simulink model "Observer"  (Simulink 8.6)
settings: Solver=ode45  StartTime=0.0  StopTime=10.0  RelTol=1e-3
values from neighbouring files (symbols this model uses):
  c1 = 5    [Parameters.m]
  c2 = 5    [Parameters.m]
  c3 = 5    [Parameters.m]
  l1 = Prm(3)    [Coriolis.m]    (also in Inertia.m; P1.m; P2.m; Parameters.m = 0.4)
  l2 = Prm(4)    [Coriolis.m]    (also in Inertia.m; P1.m; P2.m; Parameters.m = 0.3)
  m1 = Prm(1)    [Coriolis.m]    (also in Inertia.m; P1.m; Parameters.m = 1.5; Psi.m)
  m2 = Prm(2)    [Coriolis.m]    (also in Inertia.m; P1.m; P2.m; Parameters.m = 1)
  q_0 = [0;0]    [Parameters.m]
  q_dot0 = [0;0]    [Parameters.m]
  q_hat0 = [0;0]    [Parameters.m]
  r_0 = 0    [Parameters.m]
  x_hat0 = [0;0]    [Parameters.m]
  xi_0 = [0;0]    [Parameters.m]
settings Model: Creator=TOSHIBA  LastModifiedBy=TOSHIBA
settings DataIOCC: SaveFormat=StructureWithTime  SignalLoggingSaveFormat=Dataset
settings OptimizationCC: ExpressionDepthLimit=128
settings DebuggingCC: UnderspecifiedInitializationDetection=Simplified  MergeDetectMultiDrivingBlocksExec=error  SolverPrmCheckMsg=none  FcnCallInpInsideContextMsg=EnableAllAsError  StateNameClashWarn=none
settings HardwareCC: ProdBitPerPointer=64  ProdLargestAtomicFloat=Float  ProdIntDivRoundTo=Zero  ProdEndianess=LittleEndian  ProdHWDeviceType=Specified
settings GRTTargetCC: GeneratePreprocessorConditionals=Use local settings  CombineOutputUpdateFcns=on  GRTInterface=off
settings ConfigComp: CovModelRefEnable=off

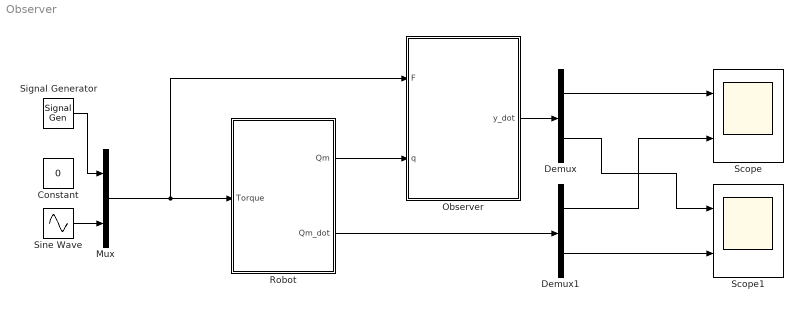
== system Observer ==
  Constant : Constant  Value=0
  Demux : Demux  Outputs=2
  Demux1 : Demux  Outputs=2
  Mux : Mux  Inputs=2
  Observer : Subsystem
  Robot : Subsystem
  Scope : Scope  NumInputPorts=2
  Scope1 : Scope  NumInputPorts=2
  Signal Generator : SignalGenerator  WaveForm=sawtooth  Amplitude=0.01  Frequency=pi  Units=rad/sec
  Sine Wave : Sin  Amplitude=0.001  Frequency=pi/1  SampleTime=0
  wires:
  Sine Wave/1 -> Mux/2
  Mux/1 -> Observer/1(F), Robot/1(Torque)
  Observer/1(y_dot) -> Demux/1
  Robot/2(Qm_dot) -> Demux1/1
  Demux/1 -> Scope/1
  Demux1/1 -> Scope/2
  Demux/2 -> Scope1/1
  Demux1/2 -> Scope1/2
  Robot/1(Qm) -> Observer/2(q)
  Signal Generator/1 -> Mux/1

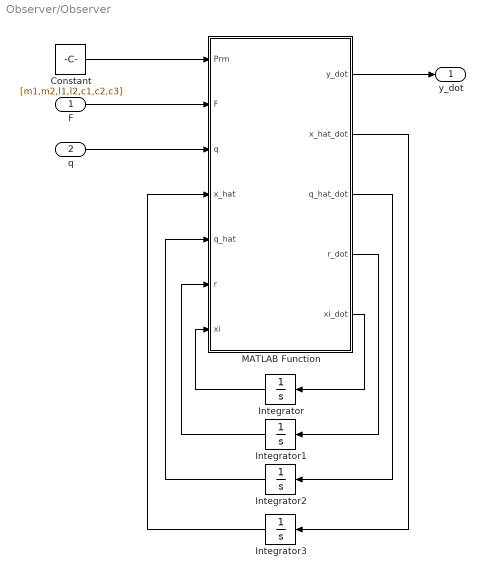
== system Observer/Observer ==
  F : Inport
  q : Inport  Port=2
  Constant : Constant  Value=[m1,m2,l1,l2,c1,c2,c3]
  Integrator : Integrator  InitialCondition=xi_0
  Integrator1 : Integrator  InitialCondition=r_0
  Integrator2 : Integrator  InitialCondition=q_hat0
  Integrator3 : Integrator  InitialCondition=x_hat0
  MATLAB Function : MATLAB Function  TreatAsAtomicUnit=on
  y_dot : Outport
  wires:
  F/1 -> MATLAB Function/2(F)
  q/1 -> MATLAB Function/3(q)
  Constant/1 -> MATLAB Function/1(Prm)
  MATLAB Function/5(xi_dot) -> Integrator/1
  Integrator/1 -> MATLAB Function/7(xi)
  Integrator1/1 -> MATLAB Function/6(r)
  MATLAB Function/4(r_dot) -> Integrator1/1
  MATLAB Function/3(q_hat_dot) -> Integrator2/1
  Integrator2/1 -> MATLAB Function/5(q_hat)
  Integrator3/1 -> MATLAB Function/4(x_hat)
  MATLAB Function/2(x_hat_dot) -> Integrator3/1
  MATLAB Function/1(y_dot) -> y_dot/1

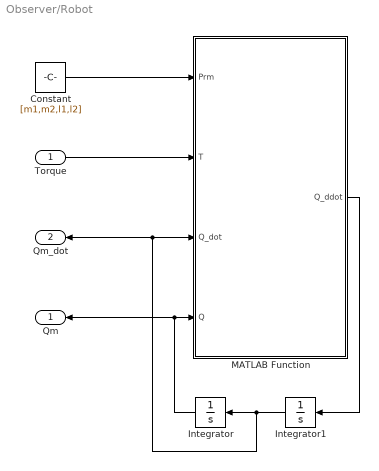
== system Observer/Robot ==
  Torque : Inport
  Constant : Constant  Value=[m1,m2,l1,l2]
  Integrator : Integrator  InitialCondition=q_0
  Integrator1 : Integrator  InitialCondition=q_dot0
  MATLAB Function : MATLAB Function  TreatAsAtomicUnit=on
  Qm : Outport
  Qm_dot : Outport  Port=2
  wires:
  Torque/1 -> MATLAB Function/2(T)
  MATLAB Function/1(Q_ddot) -> Integrator1/1
  Integrator1/1 -> MATLAB Function/3(Q_dot), Qm_dot/1, Integrator/1
  Integrator/1 -> MATLAB Function/4(Q), Qm/1
  Constant/1 -> MATLAB Function/1(Prm)

== matlab function Robot/MATLAB Function ==
  data: Prm input double; Q_ddot output double; T input double; Q_dot input double; Q input double
function Q_ddot  = RobotArm_2DOF(Prm, T, Q_dot, Q)
%#codegen
g = 9.8;
m1 = Prm(1);
m2 = Prm(2);
l1 = Prm(3);
l2 = Prm(4);

q1 = Q(1);
q2 = Q(2);
q1_dot = Q_dot(1);
q2_dot = Q_dot(2);
M11 = m2*l2^2+(m1+m2)*l1^2+2*m2*l1*l2*cos(q2);
M12 = m2*l2^2+m2*l1*l2*cos(q2);
M21 = M12;
M22 = m2*l2^2;
M = [M11, M12; M21, M22];
C11 = -2*m2*l1*l2*sin(q2)*q2_dot;
C12 = -m2*l1*l2*sin(q2)*q2_dot;
C21 = m2*l1*l2*sin(q2)*q1_dot;
C22 = 0;
C = [C11, C12; C21, C22];
g1 = m2*g*l2*sin(q1+q2)+(m1+m2)*g*l1*sin(q1);
g2 = m2*g*l2*sin(q1+q2);
G = [g1; g2];
Q_ddot = M\(T-C*Q_dot);

== matlab function Observer/MATLAB Function ==
  data: Prm input double; F input double; q input double; x_hat input double; q_hat input double; r input double; xi input double; y_dot output double; x_hat_dot output double; q_hat_dot output double; r_dot output double; xi_dot output double
function [y_dot, x_hat_dot, q_hat_dot, r_dot, xi_dot] = Observer(Prm, F, q, x_hat, q_hat, r, xi)

c1 = Prm(5);
c2 = Prm(6);
c3 = Prm(7);

psi3 = c1;

k = 4*(1+psi3);

beta = H(Prm,k,q_hat,x_hat)*q;
ex = x_hat-(xi+beta);
eq = q_hat-q;

if norm(eq)~=0
    Dq_bar = norm(Delta_q(Prm,k,q,q_hat,x_hat))/norm(eq);
else
    Dq_bar = 0;
end

if norm(ex)~=0
    Dx_bar = norm(Delta_x(Prm,q,ex))/norm(ex);
else
    Dx_bar = 0;
end

psi4 = 0.25*r^2/(1+psi3)*norm(L(Prm,q))^2*Dx_bar^2+c2;
psi5 = 0.25*r^2/(1+psi3)*norm(L(Prm,q))^2*norm(Dq_bar)^2+c3;

x_hat_dot = F+S(Prm,q,xi+beta)*(xi+beta)-0.5*r^2*norm(H(Prm,k,q_hat,x_hat))^2*norm(L(Prm,q))^2*ex-psi4*ex;
q_hat_dot = L(Prm,q)*(xi+beta)-0.5*r^2*norm(L(Prm,q))^2*eq-psi5*eq;
r_dot = -0.25*k*(r-1)+r/k*(norm(Delta_x(Prm,q,ex)*L(Prm,q))^2+norm(Delta_q(Prm,k,q,q_hat,x_hat))^2);
xi_dot = F-partial_beta_qhat(Prm,k,q,q_hat,x_hat)*q_hat_dot-partial_beta_xhat(Prm,q,q_hat)*x_hat_dot+S(Prm,q,xi+beta)*(xi+beta)-H(Prm,k,q_hat,x_hat)*L(Prm,q)*(xi+beta);

y_dot = L(Prm,q)*(xi+beta);
